simulink model "multiplexacion"  (R2023b)
settings: Solver=VariableStepAuto  StartTime=0.0  StopTime=0.1  RelTol=1e-3
values from neighbouring files (symbols this model uses):
  fc1_mux = f_portadoras(1)    [simulink_parametros.m]
  fc2_mux = f_portadoras(2)    [simulink_parametros.m]
  fc3_mux = f_portadoras(3)    [simulink_parametros.m]
  fm1_mux = 1e3    (= 1000)    [simulink_parametros.m]
  fm2_mux = 2e3    (= 2000)    [simulink_parametros.m]
  fm3_mux = 3e3    (= 3000)    [simulink_parametros.m]
  ts_mux = 1/fs_mux    (= 3.33333333333e-06)    [simulink_parametros.m]
settings Model: Creator=RomaW11  LastModifiedBy=RomaW11

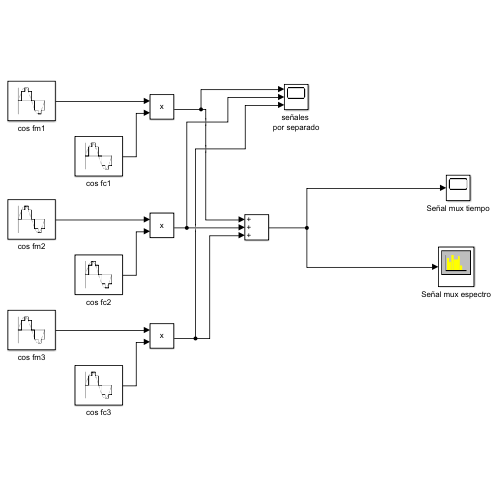
[thumbnail: Simulink's stored preview of the top-level diagram]
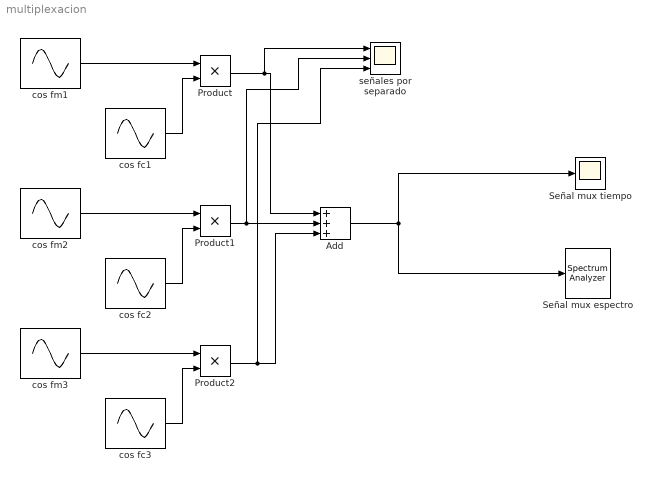
== system multiplexacion ==
  Add : Sum  Inputs=+++
  Product : Product
  Product1 : Product
  Product2 : Product
  Señal mux espectro : SpectrumAnalyzer  WindowPosition=[1.000000,1.000000,1920.000000,1057.000000,]  ScopeFrameLocation=window  SampleRateSource=Property  SampleRate=44.1e3  StartFrequency=20  StopFrequency=20e3  YLimits=[-54.57615141,25.77248512]  ShowLegend=on
  Señal mux tiempo : Scope
  cos fc1 : Sin  Frequency=fc1_mux  Phase=pi/2  SampleTime=ts_mux
  cos fc2 : Sin  Frequency=fc2_mux  Phase=pi/2  SampleTime=ts_mux
  cos fc3 : Sin  Frequency=fc3_mux  Phase=pi/2  SampleTime=ts_mux
  cos fm1 : Sin  Frequency=fm1_mux  Phase=pi/2  SampleTime=ts_mux
  cos fm2 : Sin  Frequency=fm2_mux  Phase=pi/2  SampleTime=ts_mux
  cos fm3 : Sin  Frequency=fm3_mux  Phase=pi/2  SampleTime=ts_mux
  señales por separado : Scope  NumInputPorts=3
  wires:
  cos fc1/1 -> Product/2
  cos fm1/1 -> Product/1
  Product/1 -> señales por separado/1, Add/1
  cos fc2/1 -> Product1/2
  cos fm2/1 -> Product1/1
  cos fc3/1 -> Product2/2
  cos fm3/1 -> Product2/1
  Product1/1 -> señales por separado/2, Add/2
  Product2/1 -> señales por separado/3, Add/3
  Add/1 -> Señal mux espectro/1, Señal mux tiempo/1
